simulink model "vcfp"  (R2016a)
settings: Solver=ode3  SolverMode=SingleTasking  StartTime=0.0  StopTime=0.06  FixedStep=ts  RelTol=1e-3  AbsTol=1e-6
PreLoadFcn:
  | if exist('tl_preloadfcn','file'), tl_preloadfcn(gcs,402); end
PostLoadFcn:
  | if exist('tl_postloadfcn','file'), tl_postloadfcn(gcs,402); end
InitFcn:
  | if exist('tlds_init','file'), tlds_init(gcs); end
StartFcn:
  | if exist('tlds_start','file'), tlds_start(gcs); end
StopFcn:
  | if exist('tlds_stop','file'), tlds_stop(gcs); end
values from neighbouring files (symbols this model uses):
  c12 = 1e4    (= 10000)    [vcfp_par.m]
  c23 = 1e4    (= 10000)    [vcfp_par.m]
  d1 = 0.08    [vcfp_par.m]
  d12 = 0.08    [vcfp_par.m]
  d2 = 0.08    [vcfp_par.m]
  d23 = 0.08    [vcfp_par.m]
  d3 = 0.03    [vcfp_par.m]
  J1 = 1.1e-4    (= 0.00011)    [vcfp_par.m]
  J2 = 2.6e-4    (= 0.00026)    [vcfp_par.m]
  J3 = 1.1e-4    (= 0.00011)    [vcfp_par.m]
  kE = 1    [vcfp_par.m]
  kI = 10    [vcfp_par.m]
  kM = 0.1    [vcfp_par.m]
  kr = 0.1    [vcfp_par.m]
  kx = 1e5    (= 100000)    [vcfp_par.m]
  L = 1e-4    (= 0.0001)    [vcfp_par.m]
  R = 1    [vcfp_par.m]
  ts = 0.0001    [start.m]
undefined symbols (not defined in the file or in its folder): ddv
libraries: tllib x5
PreSaveFcn:
  | if exist('tl_presavefcn','file'), tl_presavefcn(gcs); end
CloseFcn:
  | if exist('tl_closefcn','file'), tl_closefcn(gcs); end
settings Model: Tag=0  DS_PROJECTFILE=vcfp.dd  TL_MAIN_DATA={'codeopt',{'inliningthreshold',5,'assembler',1},'frameopt',{'mexargs',''},'logopt',{'plotinterval',0.02},'date',736195.49777063658}  TL_MODEL_COMMENT=The vcfp (voice coil driven flexible positioner) - model contains a 7th order plant controlled by a PID controller.  TLRevision=402  ExtModeTrigMode=oneshot  ExtModeArmWhenConnect=off  ExtModeAutoUpdateStatusClock=off  Creator=dSPACE GmbH  LastModifiedBy=db.yang
settings DataIOCC: SaveFormat=Array  SignalLoggingName=sigsOut
settings OptimizationCC: BlockReduction=off  BooleanDataType=off  OptimizeBlockIOStorage=off  BufferReuse=off  GlobalBufferReuse=off  ExpressionFolding=off  ExpressionDepthLimit=2147483647  LocalBlockOutputs=off  InitFltsAndDblsToZero=on
settings DebuggingCC: SaveWithParameterizedLinksMsg=none  UnderspecifiedInitializationDetection=Classic  MergeDetectMultiDrivingBlocksExec=none  SignalResolutionControl=TryResolveAllWithWarning  MultiTaskDSMMsg=warning  MultiTaskCondExecSysMsg=none  FcnCallInpInsideContextMsg=UseLocalSettings  BusObjectLabelMismatch=error  StateNameClashWarn=warning  StrictBusMsg=ErrorOnBusTreatedAsVector  NonBusSignalsTreatedAsBus=error
settings HardwareCC: ProdBitPerPointer=32  ProdLargestAtomicFloat=None  ProdIntDivRoundTo=Undefined  ProdEndianess=Unspecified  ProdWordSize=32  ProdHWDeviceType=32-bit Generic  TargetUnknown=on
settings ModelReferenceCC: PropagateSignalLabelsOutOfModel=off
settings RTWCC: TemplateMakefile=grt_vc.tmf
settings GRTTargetCC: TargetFcnLib=ansi_tfl_tmw.mat  ModelReferenceCompliant=off  CombineOutputUpdateFcns=off  MatFileLogging=off  GRTInterface=on
settings ConfigComp: CovModelRefEnable=Off

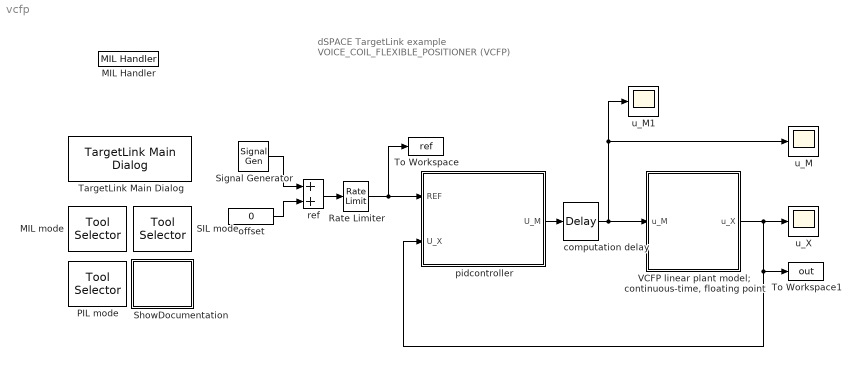
== system vcfp ==
  note: dSPACE TargetLink example
      | VOICE_COIL_FLEXIBLE_POSITIONER (VCFP)
  MIL Handler : tllib/MIL Handler  data={'date',735845.3629201852}
  MIL mode : tllib/Tool Selector  Description=MIL\nmode  data={'date',735845.3629222801}
  PIL mode : tllib/Tool Selector  Description=PIL\nmode  data={'date',735845.36292234948}
  Rate Limiter : RateLimiter  RisingSlewLimit=60  FallingSlewLimit=-60
  SIL mode : tllib/Tool Selector  Description=SIL\nmode  data={'date',735845.36292241898}
  ShowDocumentation : Subsystem
      settings: OpenFcn=if exist('tl_demos','file')==2,web([tl_get_specialfolder('TLInstallation'),'\Matlab\Demos\vcfp\html\vcfp.html']), end
      mask Display: disp('?')
  Signal Generator : SignalGenerator  WaveForm=square  Amplitude=0.1  Frequency=25
  TargetLink Main Dialog : tllib/TargetLink Main Dialog  data=[]
  To Workspace : ToWorkspace  VariableName=ref  SampleTime=-1
  To Workspace1 : ToWorkspace  VariableName=out  SampleTime=-1
  "VCFP linear plant model; continuous-time, floating point" : Subsystem
  computation delay : TransportDelay  DelayTime=ts
  offset : Constant  Value=0
  pidcontroller : Subsystem  Tag=TargetLink Simulation Frame  mask(TL_SimFrame){}
      settings: CopyFcn=if exist('tl_copyfcn','file'), tl_copyfcn(gcbh); end  NameChangeFcn=if exist('tl_framenamechangefcn','file'), tl_framenamechangefcn(gcbh); end
      settings: OpenFcn=|
      | if exist('open_tlsubsystem','file')
      |    open_tlsubsystem(gcbh);
      | else
      |    tlsubsystem = ...
      |       find_system(gcb, ...
      |       'LookUnderMasks','on', ...
      |       'FollowLinks','on', ...
      |       'Tag','MIL Subsystem');
      |    open_system(tlsubsystem);
      | end
      mask Display: disp('TargetLink\nModel-\nin-the-loop\nmode')
  ref : Sum  SaturateOnIntegerOverflow=on  InputSameDT=on  OutDataTypeStr=Inherit: Same as first input
  u_M : Scope
  u_M1 : Scope
  u_X : Scope
  wires:
  offset/1 -> ref/2
  Signal Generator/1 -> ref/1
  "VCFP linear plant model; continuous-time, floating point"/1(u_X) -> u_X/1, pidcontroller/2(U_X), To Workspace1/1
  pidcontroller/1(U_M) -> computation delay/1
  computation delay/1 -> "VCFP linear plant model; continuous-time, floating point"/1(u_M), u_M1/1, u_M/1
  ref/1 -> Rate Limiter/1
  Rate Limiter/1 -> pidcontroller/1(REF), To Workspace/1

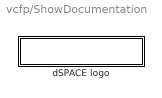
== system vcfp/ShowDocumentation ==
  dSPACE logo : Subsystem
      mask Display: image(ds_get_icon('dspace_logo_bg_white_l'))

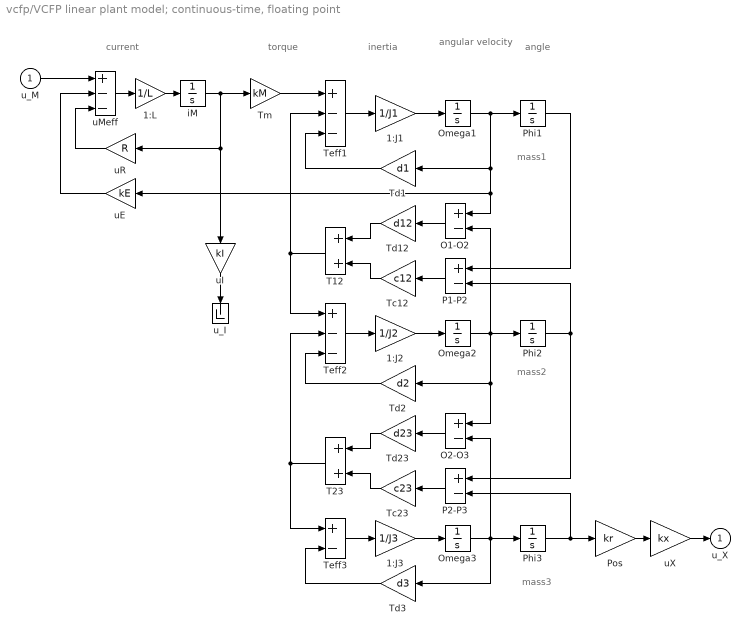
== system vcfp/VCFP linear plant model; continuous-time, floating point ==
  note: current
  note: torque
  note: inertia
  note: angular
      | velocity
  note: angle
  note: mass1
  note: mass2
  note: mass3
  u_M : Inport
  1:J1 : Gain  Gain=1/J1  SaturateOnIntegerOverflow=on  OutDataTypeStr=Inherit: Same as input  ParamDataTypeStr=Inherit: Same as input
  1:J2 : Gain  Gain=1/J2  SaturateOnIntegerOverflow=on  OutDataTypeStr=Inherit: Same as input  ParamDataTypeStr=Inherit: Same as input
  1:J3 : Gain  Gain=1/J3  SaturateOnIntegerOverflow=on  OutDataTypeStr=Inherit: Same as input  ParamDataTypeStr=Inherit: Same as input
  1:L : Gain  Gain=1/L  SaturateOnIntegerOverflow=on  OutDataTypeStr=Inherit: Same as input  ParamDataTypeStr=Inherit: Same as input
  O1-O2 : Sum  Inputs=+-  SaturateOnIntegerOverflow=on  InputSameDT=on  OutDataTypeStr=Inherit: Same as first input
  O2-O3 : Sum  Inputs=+-  SaturateOnIntegerOverflow=on  InputSameDT=on  OutDataTypeStr=Inherit: Same as first input
  Omega1 : Integrator
  Omega2 : Integrator
  Omega3 : Integrator
  P1-P2 : Sum  Inputs=+-  SaturateOnIntegerOverflow=on  InputSameDT=on  OutDataTypeStr=Inherit: Same as first input
  P2-P3 : Sum  Inputs=+-  SaturateOnIntegerOverflow=on  InputSameDT=on  OutDataTypeStr=Inherit: Same as first input
  Phi1 : Integrator
  Phi2 : Integrator
  Phi3 : Integrator
  Pos : Gain  Gain=kr  SaturateOnIntegerOverflow=on  OutDataTypeStr=Inherit: Same as input  ParamDataTypeStr=Inherit: Same as input
  T12 : Sum  SaturateOnIntegerOverflow=on  InputSameDT=on  OutDataTypeStr=Inherit: Same as first input
  T23 : Sum  SaturateOnIntegerOverflow=on  InputSameDT=on  OutDataTypeStr=Inherit: Same as first input
  Tc12 : Gain  Gain=c12  SaturateOnIntegerOverflow=on  OutDataTypeStr=Inherit: Same as input  ParamDataTypeStr=Inherit: Same as input
  Tc23 : Gain  Gain=c23  SaturateOnIntegerOverflow=on  OutDataTypeStr=Inherit: Same as input  ParamDataTypeStr=Inherit: Same as input
  Td1 : Gain  Gain=d1  SaturateOnIntegerOverflow=on  OutDataTypeStr=Inherit: Same as input  ParamDataTypeStr=Inherit: Same as input
  Td12 : Gain  Gain=d12  SaturateOnIntegerOverflow=on  OutDataTypeStr=Inherit: Same as input  ParamDataTypeStr=Inherit: Same as input
  Td2 : Gain  Gain=d2  SaturateOnIntegerOverflow=on  OutDataTypeStr=Inherit: Same as input  ParamDataTypeStr=Inherit: Same as input
  Td23 : Gain  Gain=d23  SaturateOnIntegerOverflow=on  OutDataTypeStr=Inherit: Same as input  ParamDataTypeStr=Inherit: Same as input
  Td3 : Gain  Gain=d3  SaturateOnIntegerOverflow=on  OutDataTypeStr=Inherit: Same as input  ParamDataTypeStr=Inherit: Same as input
  Teff1 : Sum  Inputs=+--  SaturateOnIntegerOverflow=on  InputSameDT=on  OutDataTypeStr=Inherit: Same as first input
  Teff2 : Sum  Inputs=+--  SaturateOnIntegerOverflow=on  InputSameDT=on  OutDataTypeStr=Inherit: Same as first input
  Teff3 : Sum  Inputs=+-  SaturateOnIntegerOverflow=on  InputSameDT=on  OutDataTypeStr=Inherit: Same as first input
  Tm : Gain  Gain=kM  SaturateOnIntegerOverflow=on  OutDataTypeStr=Inherit: Same as input  ParamDataTypeStr=Inherit: Same as input
  iM : Integrator
  uE : Gain  Gain=kE  SaturateOnIntegerOverflow=on  OutDataTypeStr=Inherit: Same as input  ParamDataTypeStr=Inherit: Same as input
  uI : Gain  Gain=kI  SaturateOnIntegerOverflow=on  OutDataTypeStr=Inherit: Same as input  ParamDataTypeStr=Inherit: Same as input
  uMeff : Sum  Inputs=+--  SaturateOnIntegerOverflow=on  InputSameDT=on  OutDataTypeStr=Inherit: Same as first input
  uR : Gain  Gain=R  SaturateOnIntegerOverflow=on  OutDataTypeStr=Inherit: Same as input  ParamDataTypeStr=Inherit: Same as input
  uX : Gain  Gain=kx  SaturateOnIntegerOverflow=on  OutDataTypeStr=Inherit: Same as input  ParamDataTypeStr=Inherit: Same as input
  u_I : Terminator
  u_X : Outport  InitialOutput=0
  wires:
  Pos/1 -> uX/1
  uI/1 -> u_I/1
  uE/1 -> uMeff/2
  uR/1 -> uMeff/3
  u_M/1 -> uMeff/1
  uX/1 -> u_X/1
  Phi3/1 -> Pos/1, P2-P3/2
  Omega3/1 -> Td3/1, O2-O3/2, Phi3/1
  Td3/1 -> Teff3/2
  T23/1 -> Teff3/1, Teff2/2
  Teff3/1 -> 1:J3/1
  1:J3/1 -> Omega3/1
  Phi2/1 -> P2-P3/1, P1-P2/2
  Td2/1 -> Teff2/3
  Omega2/1 -> Td2/1, O2-O3/1, O1-O2/2, Phi2/1
  Td23/1 -> T23/1
  Tc23/1 -> T23/2
  O2-O3/1 -> Td23/1
  P2-P3/1 -> Tc23/1
  1:J2/1 -> Omega2/1
  Teff2/1 -> 1:J2/1
  T12/1 -> Teff2/1, Teff1/2
  Phi1/1 -> P1-P2/1
  Omega1/1 -> uE/1, O1-O2/1, Td1/1, Phi1/1
  P1-P2/1 -> Tc12/1
  O1-O2/1 -> Td12/1
  Tc12/1 -> T12/2
  Td12/1 -> T12/1
  Td1/1 -> Teff1/3
  1:J1/1 -> Omega1/1
  Teff1/1 -> 1:J1/1
  Tm/1 -> Teff1/1
  iM/1 -> uI/1, uR/1, Tm/1
  1:L/1 -> iM/1
  uMeff/1 -> 1:L/1

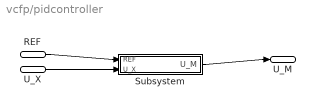
== system vcfp/pidcontroller ==
  REF : Inport  SampleTime=ts
  U_X : Inport  Port=2  SampleTime=ts
  Subsystem : Subsystem  mask(TL_Enable){}
      settings: OpenFcn=warndlg(get_param(gcb,'MaskHelp'),'Serious Warning');
      mask Help: This subsystem keeps the TargetLink subsystem (subsystem with TargetLink blocks for production code generation), and is needed for the TargetLink simulation frame to work properly. DO NOT DELETE OR MODIFY IT!
  U_M : Outport
  wires:
  REF/1 -> Subsystem/1(REF)
  U_X/1 -> Subsystem/2(U_X)
  Subsystem/1(U_M) -> U_M/1

== system vcfp/ShowDocumentation/dSPACE logo ==

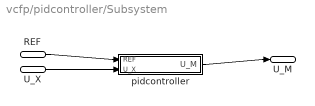
== system vcfp/pidcontroller/Subsystem ==
  REF : Inport  SampleTime=ts
  U_X : Inport  Port=2  SampleTime=ts
  pidcontroller : Subsystem  Tag=MIL Subsystem  Description=a
      settings: CopyFcn=if exist('tl_copyfcn','file'), tl_copyfcn(gcbh); end  NameChangeFcn=if exist('tl_namechangefcn','file'), tl_namechangefcn(gcbh); end  DestroyFcn=if exist('update_tl_main_dlg','file'), update_tl_main_dlg('TL_subs_display'); end
      mask Display: disp('TargetLink Subsystem')
  U_M : Outport
  wires:
  REF/1 -> pidcontroller/1(REF)
  U_X/1 -> pidcontroller/2(U_X)
  pidcontroller/1(U_M) -> U_M/1

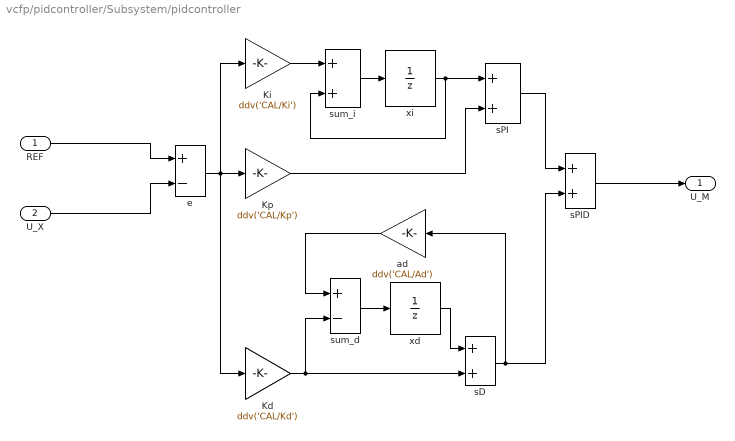
== system vcfp/pidcontroller/Subsystem/pidcontroller ==
  REF : Inport  PortDimensions=1  SampleTime=ts  mask(TL_Inport){data={'logdata',{'plotchannels',1,'loggingmode',1},'output',{'variable','DISP/REF'},'date',735845.36291979172}}
      settings: DeleteFcn=if exist('delete_tlblock','file')==2,delete_tlblock(gcbh);end  OpenFcn=if exist('tl_open_blockdlg','file')==2,tl_open_blockdlg(gcbh);else,open_system(gcbh,'parameter');end
      settings: CopyFcn=|
      | if exist('tl_reset_reviewflag','file')==2
      |     tl_reset_reviewflag(gcbh);
      | end
      | if exist('tl_check_ports','file')
      |     tl_check_ports(gcbh);
      | end
      settings: NameChangeFcn=|
      | if exist('rename_tlblock','file')==2,rename_tlblock(gcbh);end
      | if exist('tl_check_ports','file'), tl_check_ports(gcbh); end
      mask Help: eval(['if exist(''tl_online_help'',''file'') == 2, tl_online_help(''Topic'',''TL_Inport''),else, web([''jar:file:///'',matlabroot,''/help/toolbox/simulink/help.jar!/slref/' lower(get_param(gcbh,'Blocktype')) '.html''], ''-helpbrowser''),end'])
      mask Display: plot([0.2 0.35 NaN 0.65 0.8],[0 1 NaN 0 1]);
  U_X : Inport  Port=2  PortDimensions=1  SampleTime=ts  mask(TL_Inport){data={'logdata',{'plotchannels',1,'loggingmode',1},'output',{'variable','DISP/U_X'},'date',735845.36292004632}}
      settings: DeleteFcn=if exist('delete_tlblock','file')==2,delete_tlblock(gcbh);end  OpenFcn=if exist('tl_open_blockdlg','file')==2,tl_open_blockdlg(gcbh);else,open_system(gcbh,'parameter');end
      settings: CopyFcn=|
      | if exist('tl_reset_reviewflag','file')==2
      |     tl_reset_reviewflag(gcbh);
      | end
      | if exist('tl_check_ports','file')
      |     tl_check_ports(gcbh);
      | end
      settings: NameChangeFcn=|
      | if exist('rename_tlblock','file')==2,rename_tlblock(gcbh);end
      | if exist('tl_check_ports','file'), tl_check_ports(gcbh); end
      mask Help: eval(['if exist(''tl_online_help'',''file'') == 2, tl_online_help(''Topic'',''TL_Inport''),else, web([''jar:file:///'',matlabroot,''/help/toolbox/simulink/help.jar!/slref/' lower(get_param(gcbh,'Blocktype')) '.html''], ''-helpbrowser''),end'])
      mask Display: plot([0.2 0.35 NaN 0.65 0.8],[0 1 NaN 0 1]);
  Kd : Gain  Tag="Gain block of the dSPACE Fixed Point Code Generation Environment.      \\n                                                                       \\n signal is equal to the product of the input signal and the gain value:\\n\t\ty = G u"  Description=|  Gain=ddv('CAL/Kd')  mask(TL_Gain){data={'logdata',{'plotchannels',1},'output',{'lsb',2^-15},'gain',{'variable','CAL/Kd'},'date',735845.36291717598}}
      | Gain block of dSPACE TargetLink.
      | 
      | Output signal is equal to the product of the input signal and the gain value:
      |         y = G u
      settings: CopyFcn=if exist('tl_reset_reviewflag','file')==2,tl_reset_reviewflag(gcbh);end  DeleteFcn=if exist('delete_tlblock','file')==2,delete_tlblock(gcbh);end  NameChangeFcn=if exist('rename_tlblock','file')==2,rename_tlblock(gcbh);end  OpenFcn=if exist('tl_open_blockdlg','file')==2,tl_open_blockdlg(gcbh);else,open_system(gcbh,'parameter');end
      mask Help: eval(['if exist(''tl_online_help'',''file'') == 2, tl_online_help(''Topic'',''TL_Gain''),else, web([''jar:file:///'',matlabroot,''/help/toolbox/simulink/help.jar!/slref/' lower(get_param(gcbh,'Blocktype')) '.html''], ''-helpbrowser''),end'])
      mask Display: plot([0, .9, 0],[.05, .5, .95])
  Ki : Gain  Description=|  Gain=ddv('CAL/Ki')  mask(TL_Gain){data={'logdata',{'plotchannels',[]},'output',{'lsb',2^-20},'gain',{'variable','CAL/Ki'},'date',735845.36291783559}}
      | Gain block of dSPACE TargetLink.
      | 
      | Output signal is equal to the product of the input signal and the gain value:
      |         y = G u
      settings: CopyFcn=if exist('tl_reset_reviewflag','file')==2,tl_reset_reviewflag(gcbh);end  DeleteFcn=if exist('delete_tlblock','file')==2,delete_tlblock(gcbh);end  NameChangeFcn=if exist('rename_tlblock','file')==2,rename_tlblock(gcbh);end  OpenFcn=if exist('tl_open_blockdlg','file')==2,tl_open_blockdlg(gcbh);else,open_system(gcbh,'parameter');end
      mask Help: eval(['if exist(''tl_online_help'',''file'') == 2, tl_online_help(''Topic'',''TL_Gain''),else, web([''jar:file:///'',matlabroot,''/help/toolbox/simulink/help.jar!/slref/' lower(get_param(gcbh,'Blocktype')) '.html''], ''-helpbrowser''),end'])
      mask Display: plot([0, .9, 0],[.05, .5, .95])
  Kp : Gain  Tag="Gain block of the dSPACE Fixed Point Code Generation Environment.      \\n                                                                       \\n signal is equal to the product of the input signal and the gain value:\\n\t\ty = G u"  Description=|  Gain=ddv('CAL/Kp')  mask(TL_Gain){data={'logdata',{'plotchannels',[]},'output',{'lsb',2^-17},'gain',{'variable','CAL/Kp'},'date',735845.36291820602}}
      | Gain block of dSPACE TargetLink.
      | 
      | Output signal is equal to the product of the input signal and the gain value:
      |         y = G u
      settings: CopyFcn=if exist('tl_reset_reviewflag','file')==2,tl_reset_reviewflag(gcbh);end  DeleteFcn=if exist('delete_tlblock','file')==2,delete_tlblock(gcbh);end  NameChangeFcn=if exist('rename_tlblock','file')==2,rename_tlblock(gcbh);end  OpenFcn=if exist('tl_open_blockdlg','file')==2,tl_open_blockdlg(gcbh);else,open_system(gcbh,'parameter');end
      mask Help: eval(['if exist(''tl_online_help'',''file'') == 2, tl_online_help(''Topic'',''TL_Gain''),else, web([''jar:file:///'',matlabroot,''/help/toolbox/simulink/help.jar!/slref/' lower(get_param(gcbh,'Blocktype')) '.html''], ''-helpbrowser''),end'])
      mask Display: plot([0, .9, 0],[.05, .5, .95])
  ad : Gain  Tag="Gain block of the dSPACE Fixed Point Code Generation Environment.      \\n                                                                       \\n signal is equal to the product of the input signal and the gain value:\\n\t\ty = G u"  Description=|  Gain=ddv('CAL/Ad')  mask(TL_Gain){data={'logdata',{'plotchannels',[]},'output',{'lsb',2^-17},'gain',{'variable','CAL/Ad'},'date',735845.36291854165}}
      | Gain block of dSPACE TargetLink.
      | 
      | Output signal is equal to the product of the input signal and the gain value:
      |         y = G u
      settings: CopyFcn=if exist('tl_reset_reviewflag','file')==2,tl_reset_reviewflag(gcbh);end  DeleteFcn=if exist('delete_tlblock','file')==2,delete_tlblock(gcbh);end  NameChangeFcn=if exist('rename_tlblock','file')==2,rename_tlblock(gcbh);end  OpenFcn=if exist('tl_open_blockdlg','file')==2,tl_open_blockdlg(gcbh);else,open_system(gcbh,'parameter');end
      mask Help: eval(['if exist(''tl_online_help'',''file'') == 2, tl_online_help(''Topic'',''TL_Gain''),else, web([''jar:file:///'',matlabroot,''/help/toolbox/simulink/help.jar!/slref/' lower(get_param(gcbh,'Blocktype')) '.html''], ''-helpbrowser''),end'])
      mask Display: plot([0, .9, 0],[.05, .5, .95])
  e : Sum  Description=|  Inputs=+-  mask(TL_Sum){data={'logdata',{'plotchannels',1,'loggingmode',1},'output',{'variable','DISP/e','checkmin',1,'checkmax',1},'date',735845.36292115739}}
      | Sum block of dSPACE TargetLink.
      | 
      | Output signal is equal to the sum of the input signals.
      | The list of signs is specified according to conventions for Simulink Sum blocks.
      settings: CopyFcn=if exist('tl_reset_reviewflag','file')==2,tl_reset_reviewflag(gcbh);end  DeleteFcn=if exist('delete_tlblock','file')==2,delete_tlblock(gcbh);end  NameChangeFcn=if exist('rename_tlblock','file')==2,rename_tlblock(gcbh);end  OpenFcn=if exist('tl_open_blockdlg','file')==2,tl_open_blockdlg(gcbh);else,open_system(gcbh,'parameter');end
      mask Help: eval(['if exist(''tl_online_help'',''file'') == 2, tl_online_help(''Topic'',''TL_Sum''),else, web([''jar:file:///'',matlabroot,''/help/toolbox/simulink/help.jar!/slref/' lower(get_param(gcbh,'Blocktype')) '.html''], ''-helpbrowser''),end'])
      mask Display: plot([-0.05, 1.05, NaN, -0.05, 1.05],[.01, .01, NaN, .99, .99])
  sD : Sum  Tag="Sum block of the dSPACE Fixed Point Code Generation Environment.\\n                                                                \\nOutput signal is equal to the sum of the two input signals:     \\n                                                                \\n\t\ty = u1 - u2"  Description=|  mask(TL_Sum){data={'logdata',{'plotchannels',1},'output',{'lsb',2^-15},'date',735845.36292136577}}
      | Sum block of dSPACE TargetLink.
      | 
      | Output signal is equal to the sum of the input signals.
      | The list of signs is specified according to conventions for Simulink Sum blocks.
      settings: CopyFcn=if exist('tl_reset_reviewflag','file')==2,tl_reset_reviewflag(gcbh);end  DeleteFcn=if exist('delete_tlblock','file')==2,delete_tlblock(gcbh);end  NameChangeFcn=if exist('rename_tlblock','file')==2,rename_tlblock(gcbh);end  OpenFcn=if exist('tl_open_blockdlg','file')==2,tl_open_blockdlg(gcbh);else,open_system(gcbh,'parameter');end
      mask Help: eval(['if exist(''tl_online_help'',''file'') == 2, tl_online_help(''Topic'',''TL_Sum''),else, web([''jar:file:///'',matlabroot,''/help/toolbox/simulink/help.jar!/slref/' lower(get_param(gcbh,'Blocktype')) '.html''], ''-helpbrowser''),end'])
      mask Display: plot([-0.05, 1.05, NaN, -0.05, 1.05],[.01, .01, NaN, .99, .99])
  sPI : Sum  Tag="Sum block of the dSPACE Fixed Point Code Generation Environment.\\n                                                                \\nOutput signal is equal to the sum of the two input signals:     \\n                                                                \\n\t\ty = u1 - u2"  Description=|  mask(TL_Sum){data={'logdata',{'plotchannels',[]},'output',{'lsb',2^-17},'date',735845.36292157404}}
      | Sum block of dSPACE TargetLink.
      | 
      | Output signal is equal to the sum of the input signals.
      | The list of signs is specified according to conventions for Simulink Sum blocks.
      settings: CopyFcn=if exist('tl_reset_reviewflag','file')==2,tl_reset_reviewflag(gcbh);end  DeleteFcn=if exist('delete_tlblock','file')==2,delete_tlblock(gcbh);end  NameChangeFcn=if exist('rename_tlblock','file')==2,rename_tlblock(gcbh);end  OpenFcn=if exist('tl_open_blockdlg','file')==2,tl_open_blockdlg(gcbh);else,open_system(gcbh,'parameter');end
      mask Help: eval(['if exist(''tl_online_help'',''file'') == 2, tl_online_help(''Topic'',''TL_Sum''),else, web([''jar:file:///'',matlabroot,''/help/toolbox/simulink/help.jar!/slref/' lower(get_param(gcbh,'Blocktype')) '.html''], ''-helpbrowser''),end'])
      mask Display: plot([-0.05, 1.05, NaN, -0.05, 1.05],[.01, .01, NaN, .99, .99])
  sPID : Sum  Description=|  mask(TL_Sum){data={'logdata',{'plotchannels',1},'output',{'lsb',2^-15},'date',735845.36292177078}}
      | Sum block of dSPACE TargetLink.
      | 
      | Output signal is equal to the sum of the input signals.
      | The list of signs is specified according to conventions for Simulink Sum blocks.
      settings: CopyFcn=if exist('tl_reset_reviewflag','file')==2,tl_reset_reviewflag(gcbh);end  DeleteFcn=if exist('delete_tlblock','file')==2,delete_tlblock(gcbh);end  NameChangeFcn=if exist('rename_tlblock','file')==2,rename_tlblock(gcbh);end  OpenFcn=if exist('tl_open_blockdlg','file')==2,tl_open_blockdlg(gcbh);else,open_system(gcbh,'parameter');end
      mask Help: eval(['if exist(''tl_online_help'',''file'') == 2, tl_online_help(''Topic'',''TL_Sum''),else, web([''jar:file:///'',matlabroot,''/help/toolbox/simulink/help.jar!/slref/' lower(get_param(gcbh,'Blocktype')) '.html''], ''-helpbrowser''),end'])
      mask Display: plot([-0.05, 1.05, NaN, -0.05, 1.05],[.01, .01, NaN, .99, .99])
  sum_d : Sum  Description=|  Inputs=+-  mask(TL_Sum){data={'logdata',{'plotchannels',[]},'output',{'lsb',2^-15},'date',735845.36292196764}}
      | Sum block of dSPACE TargetLink.
      | 
      | Output signal is equal to the sum of the input signals.
      | The list of signs is specified according to conventions for Simulink Sum blocks.
      settings: CopyFcn=if exist('tl_reset_reviewflag','file')==2,tl_reset_reviewflag(gcbh);end  DeleteFcn=if exist('delete_tlblock','file')==2,delete_tlblock(gcbh);end  NameChangeFcn=if exist('rename_tlblock','file')==2,rename_tlblock(gcbh);end  OpenFcn=if exist('tl_open_blockdlg','file')==2,tl_open_blockdlg(gcbh);else,open_system(gcbh,'parameter');end
      mask Help: eval(['if exist(''tl_online_help'',''file'') == 2, tl_online_help(''Topic'',''TL_Sum''),else, web([''jar:file:///'',matlabroot,''/help/toolbox/simulink/help.jar!/slref/' lower(get_param(gcbh,'Blocktype')) '.html''], ''-helpbrowser''),end'])
      mask Display: plot([-0.05, 1.05, NaN, -0.05, 1.05],[.01, .01, NaN, .99, .99])
  sum_i : Sum  Tag="Sum block of the dSPACE Fixed Point Code Generation Environment.\\n                                                                \\nOutput signal is equal to the sum of the two input signals:     \\n                                                                \\n\t\ty = u1 - u2"  Description=|  mask(TL_Sum){data={'logdata',{'plotchannels',[]},'output',{'lsb',2^-19},'date',735845.36292215274}}
      | Sum block of dSPACE TargetLink.
      | 
      | Output signal is equal to the sum of the input signals.
      | The list of signs is specified according to conventions for Simulink Sum blocks.
      settings: CopyFcn=if exist('tl_reset_reviewflag','file')==2,tl_reset_reviewflag(gcbh);end  DeleteFcn=if exist('delete_tlblock','file')==2,delete_tlblock(gcbh);end  NameChangeFcn=if exist('rename_tlblock','file')==2,rename_tlblock(gcbh);end  OpenFcn=if exist('tl_open_blockdlg','file')==2,tl_open_blockdlg(gcbh);else,open_system(gcbh,'parameter');end
      mask Help: eval(['if exist(''tl_online_help'',''file'') == 2, tl_online_help(''Topic'',''TL_Sum''),else, web([''jar:file:///'',matlabroot,''/help/toolbox/simulink/help.jar!/slref/' lower(get_param(gcbh,'Blocktype')) '.html''], ''-helpbrowser''),end'])
      mask Display: plot([-0.05, 1.05, NaN, -0.05, 1.05],[.01, .01, NaN, .99, .99])
  xd : UnitDelay  Tag="Unit Delay block of the dSPACE Fixed Point Code Generation Environment.               \\n                                                                                      \\nOutput signal is equal to the input signal of the last sample step:                   \\n                                                                                      \\n\t\ty(k) = u(k-1).                                                                      \\n                                                                                      \\nIn the first sampling step, the output signal is initialized with 'initial condition':\\n                                                                                      \\n\t\ty(0) = initial condition"  Description=|  SampleTime=ts  mask(TL_UnitDelay){data={'logdata',{'plotchannels',1,'loggingmode',1},'output',{'variable','DISP/xd'},'state',{'scaling','./LocalScaling','lsb',2^-15},'date',735845.36292297451}}
      | Unit Delay block of dSPACE TargetLink.
      | 
      | Output signal is equal to the input signal of the last sample step:
      | 
      |         y(k) = u(k-1).
      | 
      | In the 1st sampling step, the output signal is initialized with 'initial condition':
      | 
      |         y(0) = initial condition
      settings: CopyFcn=if exist('tl_reset_reviewflag','file')==2,tl_reset_reviewflag(gcbh);end  DeleteFcn=if exist('delete_tlblock','file')==2,delete_tlblock(gcbh);end  NameChangeFcn=if exist('rename_tlblock','file')==2,rename_tlblock(gcbh);end  OpenFcn=if exist('tl_open_blockdlg','file')==2,tl_open_blockdlg(gcbh);else,open_system(gcbh,'parameter');end
      mask Help: eval(['if exist(''tl_online_help'',''file'') == 2, tl_online_help(''Topic'',''TL_UnitDelay''),else, web([''jar:file:///'',matlabroot,''/help/toolbox/simulink/help.jar!/slref/' lower(get_param(gcbh,'Blocktype')) '.html''], ''-helpbrowser''),end'])
      mask Display: plot([-0.05, 1.05, NaN, -0.05, 1.05],[.01, .01, NaN, .99, .99])
  xi : UnitDelay  Description=|  SampleTime=ts  mask(TL_UnitDelay){data={'logdata',{'plotchannels',1,'loggingmode',1},'output',{'variable','DISP/xi'},'state',{'scaling','./LocalScaling','lsb',2^-19},'date',735845.36292326392}}
      | Unit Delay block of dSPACE TargetLink.
      | 
      | Output signal is equal to the input signal of the last sample step:
      | 
      |         y(k) = u(k-1).
      | 
      | In the 1st sampling step, the output signal is initialized with 'initial condition':
      | 
      |         y(0) = initial condition
      settings: CopyFcn=if exist('tl_reset_reviewflag','file')==2,tl_reset_reviewflag(gcbh);end  DeleteFcn=if exist('delete_tlblock','file')==2,delete_tlblock(gcbh);end  NameChangeFcn=if exist('rename_tlblock','file')==2,rename_tlblock(gcbh);end  OpenFcn=if exist('tl_open_blockdlg','file')==2,tl_open_blockdlg(gcbh);else,open_system(gcbh,'parameter');end
      mask Help: eval(['if exist(''tl_online_help'',''file'') == 2, tl_online_help(''Topic'',''TL_UnitDelay''),else, web([''jar:file:///'',matlabroot,''/help/toolbox/simulink/help.jar!/slref/' lower(get_param(gcbh,'Blocktype')) '.html''], ''-helpbrowser''),end'])
      mask Display: plot([-0.05, 1.05, NaN, -0.05, 1.05],[.01, .01, NaN, .99, .99])
  U_M : Outport  PortDimensions=1  InitialOutput=0  mask(TL_Outport){data={'logdata',{'plotchannels',1,'loggingmode',1},'output',{'variable','DISP/U_M'},'date',735845.36292083329}}
      settings: DeleteFcn=if exist('delete_tlblock','file')==2,delete_tlblock(gcbh);end  OpenFcn=if exist('tl_open_blockdlg','file')==2,tl_open_blockdlg(gcbh);else,open_system(gcbh,'parameter');end
      settings: CopyFcn=|
      | if exist('tl_reset_reviewflag','file')==2
      |     tl_reset_reviewflag(gcbh);
      | end
      | if exist('tl_check_ports','file')
      |     tl_check_ports(gcbh);
      | end
      settings: NameChangeFcn=|
      | if exist('rename_tlblock','file')==2,rename_tlblock(gcbh);end
      | if exist('tl_check_ports','file'), tl_check_ports(gcbh); end
      mask Help: eval(['if exist(''tl_online_help'',''file'') == 2, tl_online_help(''Topic'',''TL_Outport''),else, web([''jar:file:///'',matlabroot,''/help/toolbox/simulink/help.jar!/slref/' lower(get_param(gcbh,'Blocktype')) '.html''], ''-helpbrowser''),end'])
      mask Display: plot([0.2 0.35 NaN 0.65 0.8],[0 1 NaN 0 1]);
  wires:
  Kd/1 -> sum_d/2, sD/2
  sD/1 -> ad/1, sPID/2
  sum_d/1 -> xd/1
  xd/1 -> sD/1
  ad/1 -> sum_d/1
  sPI/1 -> sPID/1
  xi/1 -> sum_i/2, sPI/1
  sum_i/1 -> xi/1
  Ki/1 -> sum_i/1
  Kp/1 -> sPI/2
  sPID/1 -> U_M/1
  U_X/1 -> e/2
  REF/1 -> e/1
  e/1 -> Ki/1, Kd/1, Kp/1
